simulink model "untitled1"  (R2018b)
settings: Solver=VariableStepAuto  StartTime=0.0  StopTime=5  RelTol=1e-3
libraries: commutil2 x1, dspsigops x1, dspquant2 x1
settings Model: Creator=nhat  LastModifiedBy=nhat

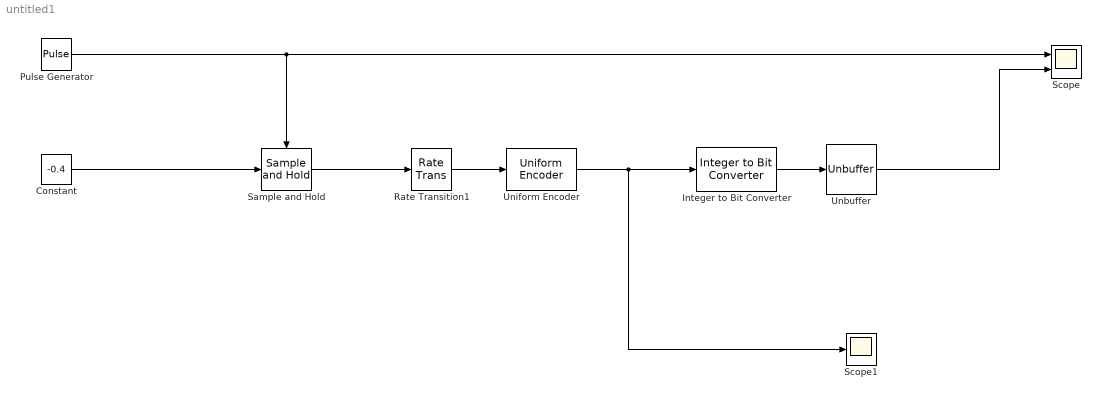
== system untitled1 ==
  Constant : Constant  Value=-0.4
  Integer to Bit Converter : commutil2/Integer to Bit Converter  nbits=8  signedInputValues=Unsigned  bitOrder=MSB first  outDtype=Inherit via internal rule
  Pulse Generator : DiscretePulseGenerator  PulseType=Time based  Period=1/8000  PulseWidth=50
  Rate Transition1 : RateTransition  OutPortSampleTime=1/8000
  Sample and Hold : dspsigops/Sample and Hold  trig=Rising edge  initCond=0  latchinput=off
  Scope : Scope  NumInputPorts=2
  Scope1 : Scope
  Unbuffer : Unbuffer
  Uniform Encoder : dspquant2/Uniform Encoder  peak=1  bits=8  otype=Unsigned integer
      settings: SourceProductName=DSP System Toolbox
  wires:
  Constant/1 -> Sample and Hold/1
  Pulse Generator/1 -> Sample and Hold/Trigger, Scope/1
  Sample and Hold/1 -> Rate Transition1/1
  Rate Transition1/1 -> Uniform Encoder/1
  Uniform Encoder/1 -> Integer to Bit Converter/1, Scope1/1
  Integer to Bit Converter/1 -> Unbuffer/1
  Unbuffer/1 -> Scope/2
